simulink model "Onboard_Autopilot_Communication"  (R2023b)
settings: Solver=FixedStepAuto  StartTime=0.0  StopTime=inf  RelTol=1e-3
undefined symbols (not defined in the file): Payload
libraries: uavmavlinklib x7, nvidiaSharedBlocks x4, nvidiaAVlib x1
settings Model: SimulationMode=external  Creator=The MathWorks, Inc.  LastModifiedBy=The MathWorks, Inc.
settings SolverCC: MaxZcPerStep=1
settings OptimizationCC: EnhancedBackFolding=on  PassReuseOutputArgsAs=Individual arguments  ZeroExternalMemoryAtStartup=off  ZeroInternalMemoryAtStartup=off  MaxStackSize=64  OptimizeBlockOrder=speed  DifferentSizesBufferReuse=on  OptimizationCustomize=off  EfficientTunableParamExpr=on
settings DebuggingCC: ParameterTunabilityLossMsg=error  UnconnectedInputMsg=warning  UnconnectedOutputMsg=warning  UnconnectedLineMsg=warning
settings HardwareCC: ProdBitPerLong=64  ProdLargestAtomicInteger=LongLong  ProdLargestAtomicFloat=Double  ProdLongLongMode=on  ProdHWDeviceType=ARM Compatible->ARM 64-bit (LP64)
settings ModelReferenceCC: EnableRefExpFcnMdlSchedulingChecks=on
settings SFSimCC: MATLABDynamicMemAlloc=off
settings RTWCC: Description=Embedded Coder  SystemTargetFile=ert.tlc  HardwareBoard=NVIDIA Jetson  TLCOptions="-aInlineSetEventsForThisBaseRateFcn=TLC_FALSE -aSuppressMultiTaskScheduler=TLC_FALSE  -aRateBasedStepFcn=0"  TemplateMakefile=ert_default_tmf  DLArmComputeVersion=19.05
settings CodeAppCC: ForceParamTrailComments=on  IgnoreCustomStorageClasses=off  MaxIdLength=63  OperatorAnnotations=on  SimulinkDataObjDesc=on  SFDataObjDesc=on  InsertBlockDesc=on

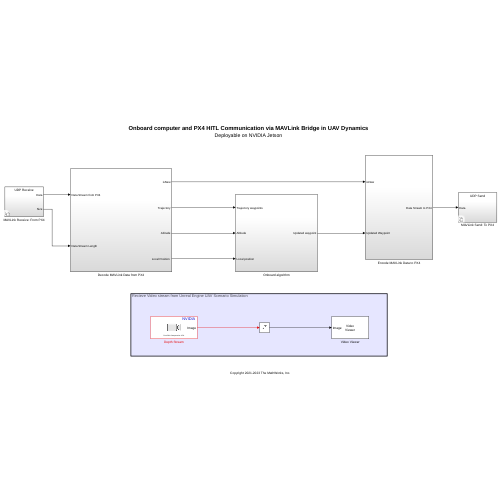
[thumbnail: Simulink's stored preview of the top-level diagram]
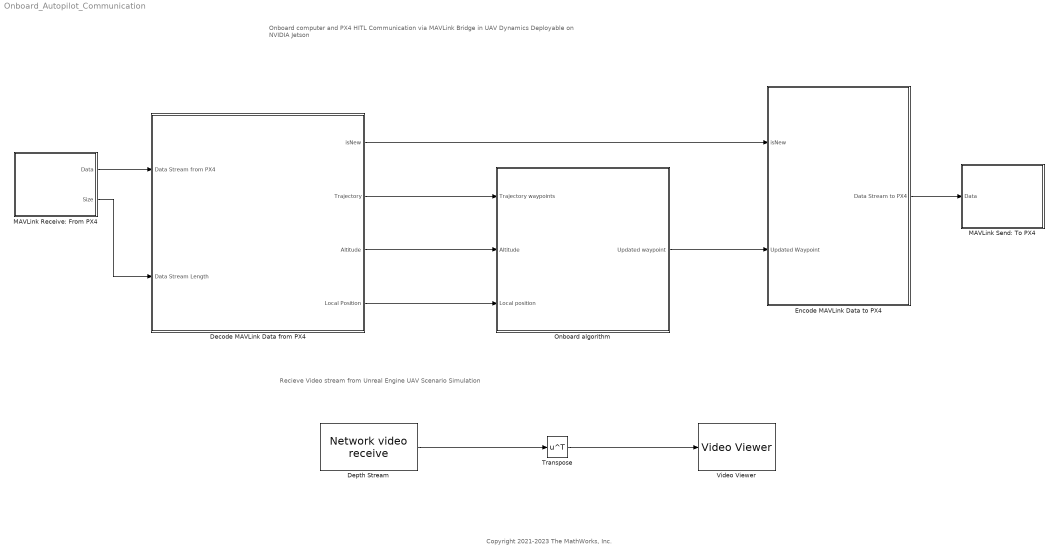
== system Onboard_Autopilot_Communication ==
  note: Recieve Video stream from Unreal Engine UAV Scenario Simulation
  note: Onboard computer and PX4 HITL Communication via MAVLink Bridge in UAV Dynamics
      | Deployable on NVIDIA Jetson
  note: Copyright 2021-2023 The MathWorks, Inc.
  Decode MAVLink Data from PX4 : Subsystem
  Depth Stream : nvidiaAVlib/Network video receive  VideoSource=Network stream  ImageSize=[360, 200]  ImageFormat=Grayscale  DeviceImageFormat=RGB  ImageSignal=Separate color signal  Decoder=VP9  VideoDeviceDecoder=H264  UseHWAcceleration=on  Port=5901  URI=rtsp://  SampleTime=0.1
  Encode MAVLink Data to PX4 : Subsystem
  MAVLink Receive: From PX4 : Subsystem  Variant=on
  MAVLink Send: To PX4 : Subsystem  Variant=on
  Onboard algorithm : Subsystem
  Transpose : Math  Operator=transpose
  Video Viewer : VideoViewer  FigPos=[1 1038 1920 938]
  wires:
  Decode MAVLink Data from PX4/4("Local Position ") -> Onboard algorithm/3(Local position)
  Decode MAVLink Data from PX4/1(isNew) -> Encode MAVLink Data to PX4/1(isNew)
  Encode MAVLink Data to PX4/1(Data Stream to PX4) -> MAVLink Send: To PX4/1(Data)
  Onboard algorithm/1(Updated waypoint) -> Encode MAVLink Data to PX4/2(Updated Waypoint)
  Decode MAVLink Data from PX4/2(Trajectory) -> Onboard algorithm/1(Trajectory waypoints)
  Decode MAVLink Data from PX4/3(Altitude) -> Onboard algorithm/2(Altitude)
  Transpose/1 -> Video Viewer/1
  Depth Stream/1 -> Transpose/1
  MAVLink Receive: From PX4/1(Data) -> Decode MAVLink Data from PX4/1(Data Stream from PX4)
  MAVLink Receive: From PX4/2(Size) -> Decode MAVLink Data from PX4/2(Data Stream Length)

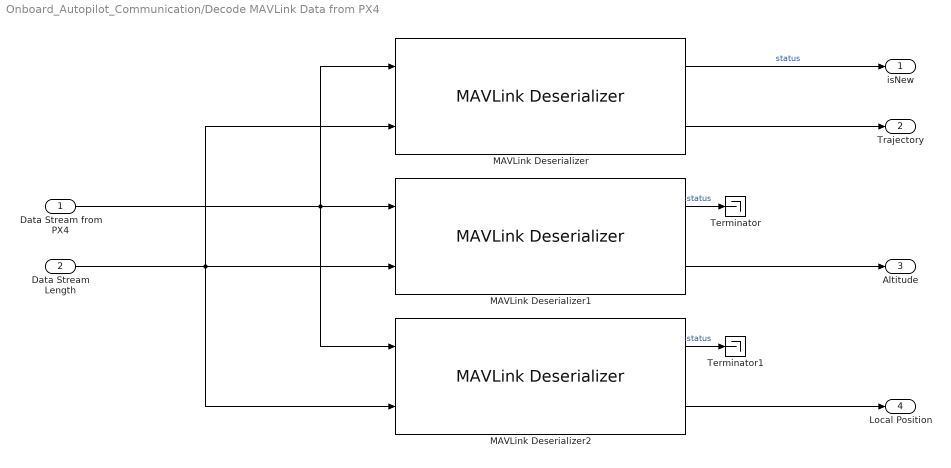
== system Onboard_Autopilot_Communication/Decode MAVLink Data from PX4 ==
  Data Stream from PX4 : Inport
  Data Stream Length : Inport  Port=2
  MAVLink Deserializer : uavmavlinklib/MAVLink Deserializer  dialectSource=Select from standard MAVLink dialects  dialect=common.xml  dialectCustom=D:\px4_110\Firmware\mavlink\include\mavlink\v2.0\message_definitions\common.xml  version=2  messageType=TRAJECTORY_REPRESENTATION_WAYPOINTS  inputDataLength=on  SystemIDFilter=off  systemID=1  ComponentIDFilter=off  componentID=1  queueMsg=off  queueMsgSize=50  dropNum=off
  MAVLink Deserializer1 : uavmavlinklib/MAVLink Deserializer  dialectSource=Select from standard MAVLink dialects  dialect=common.xml  dialectCustom=D:\px4_110\Firmware\mavlink\include\mavlink\v2.0\message_definitions\common.xml  version=2  messageType=ALTITUDE  inputDataLength=on  SystemIDFilter=off  systemID=1  ComponentIDFilter=off  componentID=1  queueMsg=off  queueMsgSize=50  dropNum=off
  MAVLink Deserializer2 : uavmavlinklib/MAVLink Deserializer  dialectSource=Select from standard MAVLink dialects  dialect=common.xml  dialectCustom=D:\px4_110\Firmware\mavlink\include\mavlink\v2.0\message_definitions\common.xml  version=2  messageType=LOCAL_POSITION_NED  inputDataLength=on  SystemIDFilter=off  systemID=1  ComponentIDFilter=off  componentID=1  queueMsg=off  queueMsgSize=50  dropNum=off
  Terminator : Terminator
  Terminator1 : Terminator
  isNew : Outport
  Trajectory : Outport  Port=2
  Altitude : Outport  Port=3
  "Local Position " : Outport  Port=4
  wires:
  Data Stream from PX4/1 -> MAVLink Deserializer/1, MAVLink Deserializer2/1, MAVLink Deserializer1/1
  MAVLink Deserializer1/1 -> Terminator/1  "status"
  MAVLink Deserializer/1 -> isNew/1  "status"
  MAVLink Deserializer1/2 -> Altitude/1
  MAVLink Deserializer2/1 -> Terminator1/1  "status"
  Data Stream Length/1 -> MAVLink Deserializer/2, MAVLink Deserializer2/2, MAVLink Deserializer1/2
  MAVLink Deserializer/2 -> Trajectory/1
  MAVLink Deserializer2/2 -> "Local Position "/1

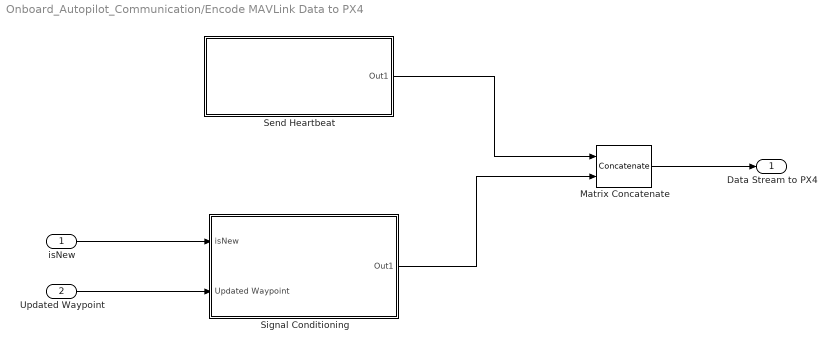
== system Onboard_Autopilot_Communication/Encode MAVLink Data to PX4 ==
  isNew : Inport
  Updated Waypoint : Inport  Port=2
  Matrix Concatenate : Concatenate  ConcatenateDimension=2
  Send Heartbeat : Subsystem
  Signal Conditioning : Subsystem
  Data Stream to PX4 : Outport
  wires:
  Signal Conditioning/1(Out1) -> Matrix Concatenate/2
  Send Heartbeat/1(Out1) -> Matrix Concatenate/1
  isNew/1 -> Signal Conditioning/1(isNew)
  Matrix Concatenate/1 -> Data Stream to PX4/1
  Updated Waypoint/1 -> Signal Conditioning/2(Updated Waypoint)

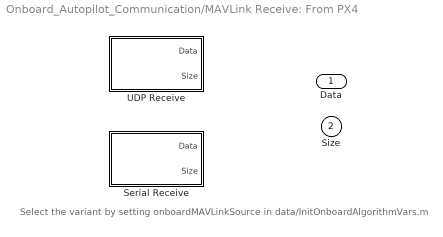
== system Onboard_Autopilot_Communication/MAVLink Receive: From PX4 ==
  note: Select the variant by setting onboardMAVLinkSource in data/InitOnboardAlgorithmVars.m
  Serial Receive : Subsystem  VariantControl=onboardMAVLinkSource == 1
  UDP Receive : Subsystem  VariantControl=onboardMAVLinkSource == 0
  Data : Outport
  Size : Outport  Port=2

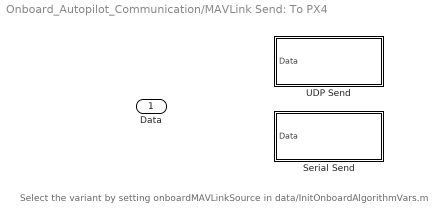
== system Onboard_Autopilot_Communication/MAVLink Send: To PX4 ==
  note: Select the variant by setting onboardMAVLinkSource in data/InitOnboardAlgorithmVars.m
  Data : Inport
  Serial Send : Subsystem  VariantControl=onboardMAVLinkSource == 1
  UDP Send : Subsystem  VariantControl=onboardMAVLinkSource == 0

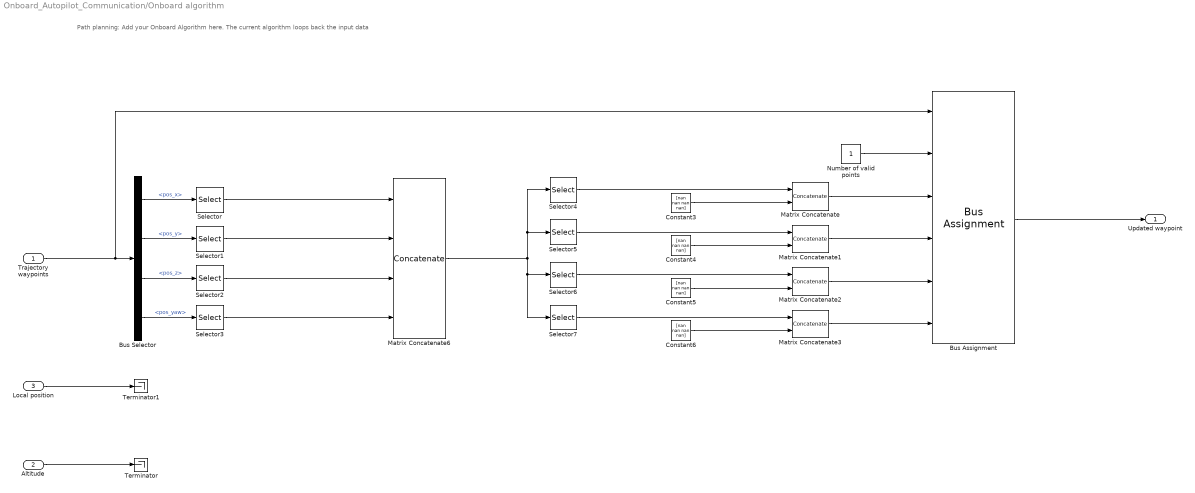
== system Onboard_Autopilot_Communication/Onboard algorithm ==
  note: Path planning: Add your Onboard Algorithm here. The current algorithm loops back the input data
  Trajectory waypoints : Inport
  Altitude : Inport  Port=2
  Local position : Inport  Port=3
  Bus Assignment : BusAssignment  AssignedSignals=Payload.valid_points,Payload.pos_x,Payload.pos_y,Payload.pos_z,Payload.pos_yaw
  Bus Selector : BusSelector  OutputSignals=Payload.pos_x,Payload.pos_y,Payload.pos_z,Payload.pos_yaw
  Constant{3..6} (4 alike) : Constant  Value=[nan nan nan nan]  OutDataTypeStr=single  SampleTime=-1
  Matrix Concatenate{,1..3} (4 alike) : Concatenate  ConcatenateDimension=2
  Matrix Concatenate6 : Concatenate  NumInputs=4  Mode=Multidimensional array
  Number of valid points : Constant  OutDataTypeStr=uint8  SampleTime=-1
  Selector{,1..3} (4 alike) : Selector  InputPortWidth=5  IndexOptions=Index vector (dialog)  Indices=2  OutputSizes=1
  Selector4 : Selector  InputPortWidth=4  IndexOptions=Index vector (dialog)  Indices=1  OutputSizes=1
  Selector5 : Selector  InputPortWidth=4  IndexOptions=Index vector (dialog)  Indices=2  OutputSizes=1
  Selector6 : Selector  InputPortWidth=4  IndexOptions=Index vector (dialog)  Indices=3  OutputSizes=1
  Selector7 : Selector  InputPortWidth=4  IndexOptions=Index vector (dialog)  Indices=4  OutputSizes=1
  Terminator : Terminator
  Terminator1 : Terminator
  Updated waypoint : Outport
  wires:
  Constant3/1 -> Matrix Concatenate/2
  Bus Assignment/1 -> Updated waypoint/1
  Matrix Concatenate/1 -> Bus Assignment/3
  Altitude/1 -> Terminator/1
  Constant4/1 -> Matrix Concatenate1/2
  Bus Selector/1 -> Selector/1  "<pos_x>"
  Selector7/1 -> Matrix Concatenate3/1
  Matrix Concatenate1/1 -> Bus Assignment/4
  Local position/1 -> Terminator1/1
  Selector6/1 -> Matrix Concatenate2/1
  Matrix Concatenate6/1 -> Selector7/1, Selector6/1, Selector4/1, Selector5/1
  Constant6/1 -> Matrix Concatenate3/2
  Selector3/1 -> Matrix Concatenate6/4
  Selector5/1 -> Matrix Concatenate1/1
  Constant5/1 -> Matrix Concatenate2/2
  Trajectory waypoints/1 -> Bus Assignment/1, Bus Selector/1
  Bus Selector/4 -> Selector3/1  "<pos_yaw>"
  Selector/1 -> Matrix Concatenate6/1
  Selector4/1 -> Matrix Concatenate/1
  Number of valid points/1 -> Bus Assignment/2
  Selector1/1 -> Matrix Concatenate6/2
  Bus Selector/2 -> Selector1/1  "<pos_y>"
  Matrix Concatenate2/1 -> Bus Assignment/5
  Matrix Concatenate3/1 -> Bus Assignment/6
  Bus Selector/3 -> Selector2/1  "<pos_z>"
  Selector2/1 -> Matrix Concatenate6/3

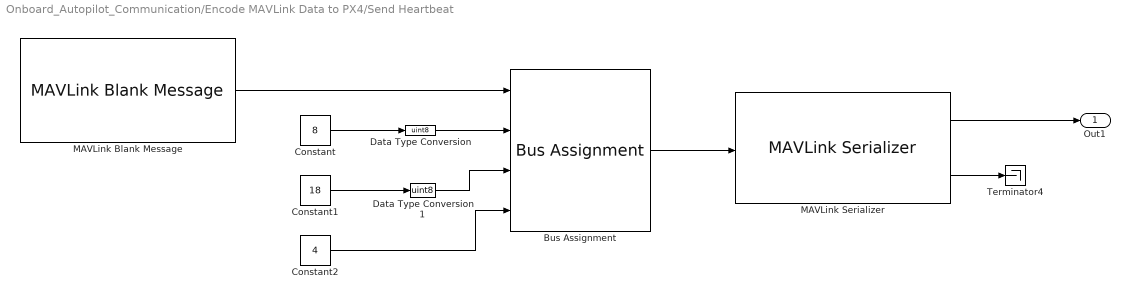
== system Onboard_Autopilot_Communication/Encode MAVLink Data to PX4/Send Heartbeat ==
  Bus Assignment : BusAssignment  AssignedSignals=Payload.autopilot,Payload.type,Payload.system_status
  Constant : Constant  Value=8  SampleTime=-1
  Constant1 : Constant  Value=18  SampleTime=-1
  Constant2 : Constant  Value=4  OutDataTypeStr=uint8  SampleTime=-1
  Data Type Conversion : DataTypeConversion  OutDataTypeStr=uint8  SaturateOnIntegerOverflow=off  RndMeth=Floor
  Data Type Conversion1 : DataTypeConversion  OutDataTypeStr=uint8  SaturateOnIntegerOverflow=off  RndMeth=Floor
  MAVLink Blank Message : uavmavlinklib/MAVLink Blank Message  dialectSource=Select from standard MAVLink dialects  dialect=common.xml  dialectCustom=D:\px4_110\Firmware\mavlink\include\mavlink\v2.0\message_definitions\common.xml  version=2  messageType=HEARTBEAT  SystemID=1  ComponentID=196  SampleTime=-1
  MAVLink Serializer : uavmavlinklib/MAVLink Serializer  dialectSource=Select from standard MAVLink dialects  dialect=common.xml  dialectCustom=D:\px4_110\Firmware\mavlink\include\mavlink\v2.0\message_definitions\common.xml  version=2  messageType=HEARTBEAT
  Terminator4 : Terminator
  Out1 : Outport
  wires:
  Bus Assignment/1 -> MAVLink Serializer/1
  Constant/1 -> Data Type Conversion/1
  MAVLink Serializer/1 -> Out1/1
  Data Type Conversion1/1 -> Bus Assignment/3
  Data Type Conversion/1 -> Bus Assignment/2
  MAVLink Serializer/2 -> Terminator4/1
  Constant1/1 -> Data Type Conversion1/1
  MAVLink Blank Message/1 -> Bus Assignment/1
  Constant2/1 -> Bus Assignment/4

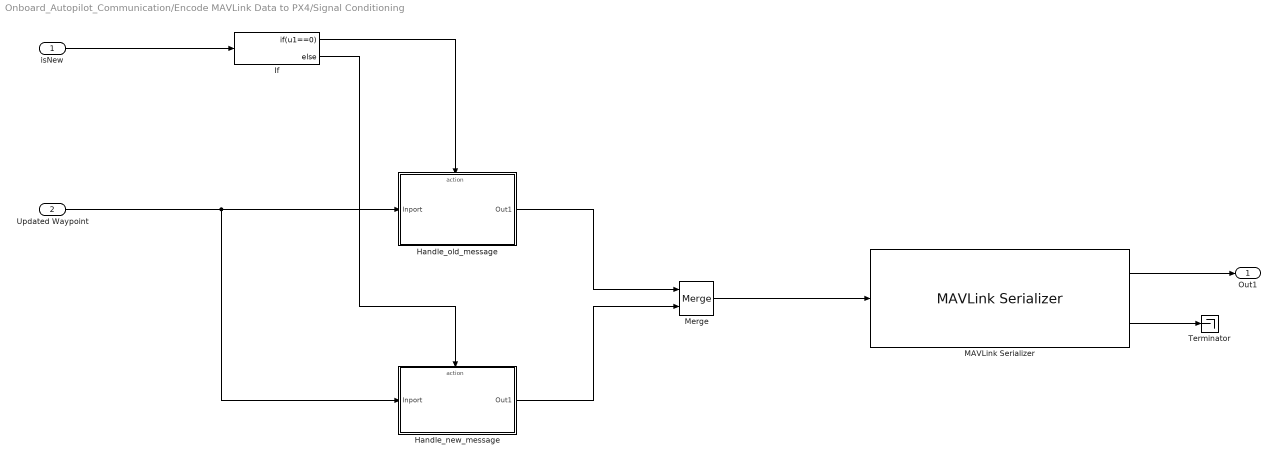
== system Onboard_Autopilot_Communication/Encode MAVLink Data to PX4/Signal Conditioning ==
  isNew : Inport
  Updated Waypoint : Inport  Port=2
  Handle_new_message : Subsystem  TreatAsAtomicUnit=on
  Handle_old_message : Subsystem  TreatAsAtomicUnit=on
  If : If  IfExpression=u1==0
  MAVLink Serializer : uavmavlinklib/MAVLink Serializer  dialectSource=Select from standard MAVLink dialects  dialect=common.xml  dialectCustom=D:\px4_110\Firmware\mavlink\include\mavlink\v2.0\message_definitions\common.xml  version=2  messageType=TRAJECTORY_REPRESENTATION_WAYPOINTS
  Merge : Merge
  Terminator : Terminator
  Out1 : Outport
  wires:
  MAVLink Serializer/2 -> Terminator/1
  MAVLink Serializer/1 -> Out1/1
  isNew/1 -> If/1
  Updated Waypoint/1 -> Handle_new_message/1(Inport), Handle_old_message/1(Inport)
  If/2 -> Handle_new_message/Action
  Handle_old_message/1(Out1) -> Merge/1
  Merge/1 -> MAVLink Serializer/1
  Handle_new_message/1(Out1) -> Merge/2
  If/1 -> Handle_old_message/Action

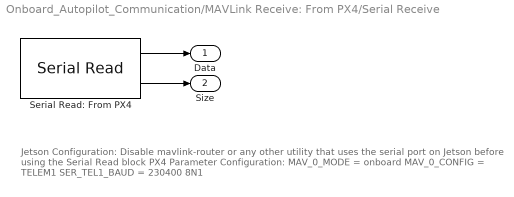
== system Onboard_Autopilot_Communication/MAVLink Receive: From PX4/Serial Receive ==
  note: Jetson Configuration:
      | Disable mavlink-router or any other utility that uses the serial port on Jetson before using the Serial Read block
      |
      | PX4 Parameter Configuration:
      | MAV_0_MODE = onboard
      | MAV_0_CONFIG = TELEM1
      | SER_TEL1_BAUD = 230400 8N1
  Serial Read: From PX4 : nvidiaSharedBlocks/Serial Read  board=Pi 3 Model B  SCIModule_=/dev/ttyTHS0  Baudrate_=230400  Parity=None  StopBits_=1  HardwareFlowControl=None  ByteOrder=LittleEndian  DataLength=4096  DataType=uint8  OutputStatus=on  SampleTime=0.1  blockPlatform=NVIDIA  BlockingMode=off  Timeout=5  outputPartialData=on
      settings: LibrarySourceBlock=nvidiaCommlib/Serial Read
  Data : Outport
  Size : Outport  Port=2
  wires:
  Serial Read: From PX4/1 -> Data/1
  Serial Read: From PX4/2 -> Size/1

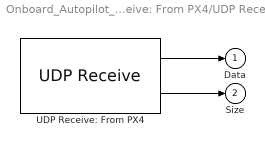
== system Onboard_Autopilot_Communication/MAVLink Receive: From PX4/UDP Receive ==
  UDP Receive: From PX4 : nvidiaSharedBlocks/UDP Receive  localURL='0.0.0.0'  localPort=14540  remoteURL='0.0.0.0'  remotePort=-1  recvBufferSize=8192  signalDatatype=uint8  dims=512  isVarSize=off  showBlockingTime=off  blockingTime=0  sampletime=0.1  blockPlatform=NVIDIA
  Data : Outport
  Size : Outport  Port=2
  wires:
  UDP Receive: From PX4/1 -> Data/1
  UDP Receive: From PX4/2 -> Size/1

== system Onboard_Autopilot_Communication/MAVLink Send: To PX4/Serial Send ==
  note: Disable mavlink-router or any other utility that uses the serial port on Jetson before using the Serial Write block
  Data : Inport
  Serial Write: To PX4 : nvidiaSharedBlocks/Serial Write  board=Pi 3 Model B  SCIModule_=/dev/ttyTHS0  Baudrate_=230400  Parity=None  StopBits_=1  HardwareFlowControl=None  ByteOrder=LittleEndian  OutputStatus=off  blockPlatform=NVIDIA
      settings: LibrarySourceBlock=nvidiaCommlib/Serial Write
  wires:
  Data/1 -> Serial Write: To PX4/1

== system Onboard_Autopilot_Communication/MAVLink Send: To PX4/UDP Send ==
  Data : Inport
  "UDP Send : To PX4" : nvidiaSharedBlocks/UDP Send  remoteURL='172.19.98.115'  remotePort=14580  localURL='0.0.0.0'  localPortSource=Automatically determine  localPort=-1  sampletime=-1  blockPlatform=NVIDIA  separateLengthPort=0
  wires:
  Data/1 -> "UDP Send : To PX4"/1

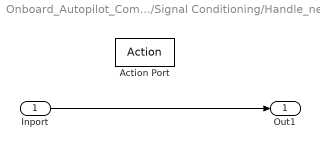
== system Onboard_Autopilot_Communication/Encode MAVLink Data to PX4/Signal Conditioning/Handle_new_message ==
  Inport : Inport
  Action Port : ActionPort  ActionPortLabel=else
  Out1 : Outport
  wires:
  Inport/1 -> Out1/1

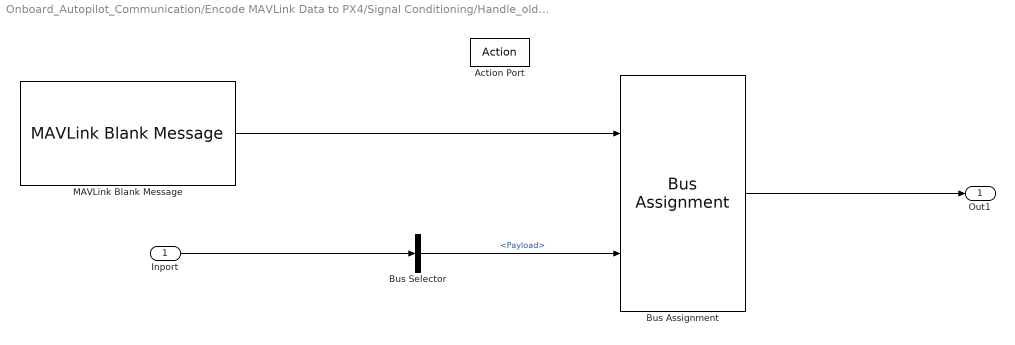
== system Onboard_Autopilot_Communication/Encode MAVLink Data to PX4/Signal Conditioning/Handle_old_message ==
  Inport : Inport
  Action Port : ActionPort  ActionPortLabel=if(u1==0)
  Bus Assignment : BusAssignment  AssignedSignals=Payload
  Bus Selector : BusSelector  OutputSignals=Payload
  MAVLink Blank Message : uavmavlinklib/MAVLink Blank Message  dialectSource=Select from standard MAVLink dialects  dialect=common.xml  dialectCustom=D:\px4_110\Firmware\mavlink\include\mavlink\v2.0\message_definitions\common.xml  version=2  messageType=TRAJECTORY_REPRESENTATION_WAYPOINTS  SystemID=1  ComponentID=196  SampleTime=-1
  Out1 : Outport
  wires:
  MAVLink Blank Message/1 -> Bus Assignment/1
  Bus Assignment/1 -> Out1/1
  Inport/1 -> Bus Selector/1
  Bus Selector/1 -> Bus Assignment/2  "<Payload>"
